simulink model "Basic_DMT"  (R2014b)
settings: Solver=FixedStepDiscrete  SolverMode=SingleTasking  StartTime=0.0  StopTime=25e-6-14e-9*24  RelTol=1e-3
PreLoadFcn:
  | userName = getenv('UserName');
  | 
  | if strcmp(userName,'Tim')
  | cd C:\Users\Tim\Documents\GitHub\MA_1\Basic_DMT
  | else
  | cd C:\Users\Tim-UML\Documents\GitHub\MA_1\Basic_DMT
  | end
InitFcn:
  | userName = getenv('UserName');
  | 
  | if strcmp(userName,'Tim')
  | cd C:\Users\Tim\Documents\GitHub\MA_1\Basic_DMT
  | else
  | cd C:\Users\Tim-UML\Documents\GitHub\MA_1\Basic_DMT
  | end
values from neighbouring files (symbols this model uses):
  a0 = 0.21194908595403703    (= 0.211949085954)    [initScript.m]
  a1 = 0.576101828091926    (= 0.576101828092)    [initScript.m]
  a2 = a0    (= 0.211949085954)    [initScript.m]
  beta = 1    [initScript.m]
  bitPerSymb = 4    [initScript.m]
  chanDownFact = Tchan/SystemPeriod    [initScript.m]
  fftLen = 16    [initScript.m]
  fftLenActive = fftLenDMT    (= 32)    [initScript.m]
  fftLenDMT = 2*fftLen    (= 32)    [initScript.m]
  GI_Active = GI_LenDMT    (= 0)    [initScript.m]
  GI_Len = 0    [initScript.m]
  GI_LenDMT = 0    [initScript.m]
  M = log2(fftLen)    [initScript.m]
  sysgenSystemPeriod = 4e-9    (= 4e-09)    [initScript.m]
  SystemPeriod = 4e-9    (= 4e-09)    [initScript.m]
  upsampleFactor = 1    [initScript.m]
  usedSubCar = 14    [initScript.m]
undefined symbols (not defined in the file or in its folder): bitCount, get, modu_mode, Tb, Ts
libraries: xbsIndex_r4 x822, commdigbbndam3 x59, simulink x42, dspsigops x7, commrandsrc2 x6, dspbuff3 x4, dspxfrm3 x3, dspswit3 x2, commseqgen2 x1, dsparch4 x1, commutil2 x1, dspsnks4 x1
(part 7 of 10)

== system Basic_DMT/IFFTaPIS/Guard_Interval/Set_GI_DMT ==
  note: 13
  note: max count == fftLen+GI_Len-1?
      | initial value== fftLen-1?
  In1 : Inport
  Complex to Real-Imag : ComplexToRealImag
  Constant : Constant
  Counter : dspswit3/Counter  Direction=Up  CountEvent=Free running  CounterSize=User defined  MaxCount=fftLenDMT+GI_LenDMT-1  InitialCount=32  Output=Count  HitValue=5  ResetInput=off  SamplesPerFrame=1  Ts=Tb*usedSubCar*bitPerSymb/fftLenDMT*beta  CntDtype=double  HitDtype=Logical
  Delay : Delay  DelayLength=53  InitialCondition=0
  Demux : Demux  Outputs=32
  Fcn : Fcn  Expr=u>fftLenDMT-1
  From Workspace : FromWorkspace  Commented=on  VariableName=sig_dmt_GI  SampleTime=1.12e-6  Interpolate=off  OutputAfterFinalValue=Setting to zero
  Mux : Mux  Inputs=40
  Scope : Scope  NumInputPorts=2
      settings: YMin=-5~-5  YMax=5~5  SaveName=ScopeData31
  Spectrum Analyzer1 : SpectrumAnalyzer  Commented=on
  Terminator : Terminator
  To Workspace : ToWorkspace  Commented=on  VariableName=sig_dmt_GI  SaveFormat=Structure  SampleTime=-1
  Unbuffer1 : Unbuffer  SampleBasedProcessing=Same as frame based
  Out1 : Outport
  pop : Outport  Port=2
  wires:
  In1/1 -> Demux/1
  Fcn/1 -> Scope/2
  Mux/1 -> To Workspace/1, Unbuffer1/1
  Complex to Real-Imag/1 -> Scope/1
  Complex to Real-Imag/2 -> Terminator/1
  Counter/1 -> Fcn/1
  Delay/1 -> Out1/1
  Demux/32 -> Mux/8, Mux/40
  Demux/31 -> Mux/7, Mux/39
  Demux/30 -> Mux/6, Mux/38
  Demux/29 -> Mux/5, Mux/37
  Demux/28 -> Mux/4, Mux/36
  Demux/27 -> Mux/3, Mux/35
  Demux/26 -> Mux/2, Mux/34
  Demux/25 -> Mux/1, Mux/33
  Demux/24 -> Mux/32
  Demux/23 -> Mux/31
  Demux/22 -> Mux/30
  Demux/21 -> Mux/29
  Demux/20 -> Mux/28
  Demux/19 -> Mux/27
  Demux/18 -> Mux/26
  Demux/17 -> Mux/25
  Demux/16 -> Mux/24
  Demux/15 -> Mux/23
  Demux/14 -> Mux/22
  Demux/13 -> Mux/21
  Demux/12 -> Mux/20
  Demux/11 -> Mux/19
  Demux/10 -> Mux/18
  Demux/9 -> Mux/17
  Demux/8 -> Mux/16
  Demux/7 -> Mux/15
  Demux/6 -> Mux/14
  Demux/5 -> Mux/13
  Demux/4 -> Mux/12
  Demux/3 -> Mux/11
  Demux/2 -> Mux/10
  Demux/1 -> Mux/9
  Unbuffer1/1 -> Delay/1, Complex to Real-Imag/1
  From Workspace/1 -> Spectrum Analyzer1/1
  Constant/1 -> pop/1

== system Basic_DMT/IFFTaPIS/Guard_Interval/Set_GI_OFDM ==
  note: 13
  note: max count == fftLen+GI_Len-1?
      | initial value== fftLen-1?
  note: 33
  In1 : Inport
  Complex to Real-Imag : ComplexToRealImag  Commented=on
  Complex to Real-Imag1 : ComplexToRealImag
  Complex to Real-Imag2 : ComplexToRealImag
  Counter : dspswit3/Counter  Commented=on  Direction=Up  CountEvent=Free running  CounterSize=User defined  MaxCount=19  InitialCount=16  Output=Count  HitValue=5  ResetInput=off  SamplesPerFrame=1  Ts=Tb*usedSubCar*bitPerSymb/fftLen*beta  CntDtype=double  HitDtype=Logical
  Data Store Memory : DataStoreMemory  DataStoreName=state  OutDataTypeStr=double
  Data Store Memory2 : DataStoreMemory  DataStoreName=loopCount  OutDataTypeStr=double
  Delay : Delay  Commented=on  DelayLength=33  InitialCondition=0
  Delay{1..17} (17 alike) : Delay  DelayLength=1  InitialCondition=0
  Delay18 : Delay  Commented=through  DelayLength=33  InitialCondition=0
  Delay19 : Delay  Commented=through  DelayLength=33  InitialCondition=0
  Demux1 : Demux  Commented=on  Outputs=16
  Fcn : Fcn  Commented=on  Expr=u>fftLen-1
  MATLAB Function : MATLAB Function  TreatAsAtomicUnit=on  SystemSampleTime=SystemPeriod*bitPerSymb*usedSubCar/fftLenActive
  Mux1 : Mux  Commented=on  Inputs=20
  Scope : Scope  Commented=on  NumInputPorts=2
      settings: YMin=-5~-5  YMax=5~5  SaveName=ScopeData31
  Scope1 : Scope  NumInputPorts=3
      settings: YMin=-5~-5~-5  YMax=5~5~5  SaveName=ScopeData69
  Terminator : Terminator  Commented=on
  Unbuffer1 : Unbuffer  Commented=on  SampleBasedProcessing=Same as frame based
  Unbuffer2 : Unbuffer  SampleBasedProcessing=Same as frame based
  Out1 : Outport
  pop : Outport  Port=2
  wires:
  Fcn/1 -> Scope/2
  Unbuffer1/1 -> Complex to Real-Imag/1, Delay/1
  Complex to Real-Imag/1 -> Scope/1
  Complex to Real-Imag/2 -> Terminator/1
  Counter/1 -> Fcn/1
  Demux1/8 -> Mux1/12
  Demux1/7 -> Mux1/11
  Demux1/6 -> Mux1/10
  Demux1/5 -> Mux1/9
  Demux1/4 -> Mux1/8
  Demux1/3 -> Mux1/7
  Demux1/2 -> Mux1/6
  Demux1/1 -> Mux1/5
  Mux1/1 -> Unbuffer1/1
  Demux1/9 -> Mux1/13
  Demux1/10 -> Mux1/14
  Demux1/11 -> Mux1/15
  Demux1/12 -> Mux1/16
  Demux1/13 -> Mux1/1, Mux1/17
  Demux1/14 -> Mux1/2, Mux1/18
  Demux1/15 -> Mux1/3, Mux1/19
  Demux1/16 -> Mux1/4, Mux1/20
  MATLAB Function/2(o1) -> Delay1/1
  MATLAB Function/3(o2) -> Delay2/1
  MATLAB Function/4(o3) -> Delay3/1
  MATLAB Function/5(o4) -> Delay4/1
  MATLAB Function/9(o8) -> Delay8/1
  MATLAB Function/8(o7) -> Delay7/1
  MATLAB Function/7(o6) -> Delay6/1
  MATLAB Function/6(o5) -> Delay5/1
  MATLAB Function/13(o12) -> Delay12/1
  MATLAB Function/12(o11) -> Delay11/1
  MATLAB Function/11(o10) -> Delay10/1
  MATLAB Function/10(o9) -> Delay9/1
  MATLAB Function/14(o13) -> Delay13/1
  MATLAB Function/15(o14) -> Delay14/1
  MATLAB Function/16(o15) -> Delay15/1
  MATLAB Function/17(o16) -> Delay16/1
  Delay16/1 -> MATLAB Function/17(i16)
  Delay15/1 -> MATLAB Function/16(i15)
  Delay14/1 -> MATLAB Function/15(i14)
  Delay13/1 -> MATLAB Function/14(i13)
  Delay12/1 -> MATLAB Function/13(i12)
  Delay11/1 -> MATLAB Function/12(i11)
  Delay10/1 -> MATLAB Function/11(i10)
  Delay9/1 -> MATLAB Function/10(i9)
  Delay8/1 -> MATLAB Function/9(i8)
  Delay7/1 -> MATLAB Function/8(i7)
  Delay6/1 -> MATLAB Function/7(i6)
  Delay5/1 -> MATLAB Function/6(i5)
  Delay4/1 -> MATLAB Function/5(i4)
  Delay3/1 -> MATLAB Function/4(i3)
  Delay2/1 -> MATLAB Function/3(i2)
  Delay1/1 -> MATLAB Function/2(i1)
  Unbuffer2/1 -> Delay17/1
  In1/1 -> Unbuffer2/1
  MATLAB Function/18(pop) -> Scope1/3, Delay19/1
  Complex to Real-Imag1/1 -> Scope1/2
  Complex to Real-Imag2/1 -> Scope1/1
  Delay17/1 -> Complex to Real-Imag2/1, MATLAB Function/1(inp)
  MATLAB Function/1(out) -> Delay18/1, Complex to Real-Imag1/1
  Delay18/1 -> Out1/1
  Delay19/1 -> pop/1

== system Basic_DMT/IFFTaPIS/upsample/upsample_No ==
  In1 : Inport
  Out1 : Outport
  wires:
  In1/1 -> Out1/1

== system Basic_DMT/IFFTaPIS/upsample/upsample_yes ==
  In1 : Inport
  Complex to Real-Imag : ComplexToRealImag
  Complex to Real-Imag1 : ComplexToRealImag
  Scope3 : Scope  NumInputPorts=4
      settings: YMin=-10~-8~-5~-5  YMax=8~8~5~5  SaveName=ScopeData38
  Unbuffer : Unbuffer  SampleBasedProcessing=Same as frame based
  Unbuffer1 : Unbuffer  SampleBasedProcessing=Same as frame based
  Upsample1 : dspsigops/Upsample  N=upsampleFactor  phase=0  InputProcessing=Columns as channels (frame based)  RateOptions=Enforce single-rate processing  ic=0  mode=Unused parameter value
  Out1 : Outport
  wires:
  In1/1 -> Unbuffer1/1, Upsample1/1
  Upsample1/1 -> Unbuffer/1, Out1/1
  Complex to Real-Imag/1 -> Scope3/1
  Complex to Real-Imag/2 -> Scope3/3
  Complex to Real-Imag1/1 -> Scope3/2
  Complex to Real-Imag1/2 -> Scope3/4
  Unbuffer/1 -> Complex to Real-Imag/1
  Unbuffer1/1 -> Complex to Real-Imag1/1

== system Basic_DMT/Modulation/Bit_Mapping_P1/16_QAM ==
  In1 : Inport
  Enable : EnablePort
  Rect_QAM_Mod : commdigbbndam3/Rectangular QAM Modulator Baseband  M=16  InType=Bit  Enc=Gray  Mapping=[0:15]  PowType=Min. distance between symbols  MinDist=2  AvgPow=1  PeakPow=1  Ph=0  outDtype=double  outWordLen=16  outUDDataType=sfix(16)  outFracLenMode=User-defined  outFracLen=13
  Out1 : Outport
  wires:
  Rect_QAM_Mod/1 -> Out1/1
  In1/1 -> Rect_QAM_Mod/1

== system Basic_DMT/Modulation/Bit_Mapping_P1/256_QAM ==
  In1 : Inport
  Enable : EnablePort
  Rect_QAM_Mod : commdigbbndam3/Rectangular QAM Modulator Baseband  M=16  InType=Bit  Enc=Gray  Mapping=[0:15]  PowType=Min. distance between symbols  MinDist=2  AvgPow=1  PeakPow=1  Ph=0  outDtype=double  outWordLen=16  outUDDataType=sfix(16)  outFracLenMode=User-defined  outFracLen=13
  Out1 : Outport
  wires:
  Rect_QAM_Mod/1 -> Out1/1
  In1/1 -> Rect_QAM_Mod/1

== system Basic_DMT/Modulation/Bit_Mapping_P10/16_QAM ==
  In1 : Inport
  Enable : EnablePort
  Rect_QAM_Mod : commdigbbndam3/Rectangular QAM Modulator Baseband  M=16  InType=Bit  Enc=Gray  Mapping=[0:15]  PowType=Min. distance between symbols  MinDist=2  AvgPow=1  PeakPow=1  Ph=0  outDtype=double  outWordLen=16  outUDDataType=sfix(16)  outFracLenMode=User-defined  outFracLen=13
  Out1 : Outport
  wires:
  Rect_QAM_Mod/1 -> Out1/1
  In1/1 -> Rect_QAM_Mod/1

== system Basic_DMT/Modulation/Bit_Mapping_P10/256_QAM ==
  In1 : Inport
  Enable : EnablePort
  Rect_QAM_Mod : commdigbbndam3/Rectangular QAM Modulator Baseband  M=16  InType=Bit  Enc=Gray  Mapping=[0:15]  PowType=Min. distance between symbols  MinDist=2  AvgPow=1  PeakPow=1  Ph=0  outDtype=double  outWordLen=16  outUDDataType=sfix(16)  outFracLenMode=User-defined  outFracLen=13
  Out1 : Outport
  wires:
  Rect_QAM_Mod/1 -> Out1/1
  In1/1 -> Rect_QAM_Mod/1

== system Basic_DMT/Modulation/Bit_Mapping_P11/16_QAM ==
  In1 : Inport
  Enable : EnablePort
  Rect_QAM_Mod : commdigbbndam3/Rectangular QAM Modulator Baseband  M=16  InType=Bit  Enc=Gray  Mapping=[0:15]  PowType=Min. distance between symbols  MinDist=2  AvgPow=1  PeakPow=1  Ph=0  outDtype=double  outWordLen=16  outUDDataType=sfix(16)  outFracLenMode=User-defined  outFracLen=13
  Out1 : Outport
  wires:
  Rect_QAM_Mod/1 -> Out1/1
  In1/1 -> Rect_QAM_Mod/1

== system Basic_DMT/Modulation/Bit_Mapping_P11/256_QAM ==
  In1 : Inport
  Enable : EnablePort
  Rect_QAM_Mod : commdigbbndam3/Rectangular QAM Modulator Baseband  M=16  InType=Bit  Enc=Gray  Mapping=[0:15]  PowType=Min. distance between symbols  MinDist=2  AvgPow=1  PeakPow=1  Ph=0  outDtype=double  outWordLen=16  outUDDataType=sfix(16)  outFracLenMode=User-defined  outFracLen=13
  Out1 : Outport
  wires:
  Rect_QAM_Mod/1 -> Out1/1
  In1/1 -> Rect_QAM_Mod/1

== system Basic_DMT/Modulation/Bit_Mapping_P12/16_QAM ==
  In1 : Inport
  Enable : EnablePort
  Rect_QAM_Mod : commdigbbndam3/Rectangular QAM Modulator Baseband  M=16  InType=Bit  Enc=Gray  Mapping=[0:15]  PowType=Min. distance between symbols  MinDist=2  AvgPow=1  PeakPow=1  Ph=0  outDtype=double  outWordLen=16  outUDDataType=sfix(16)  outFracLenMode=User-defined  outFracLen=13
  Out1 : Outport
  wires:
  Rect_QAM_Mod/1 -> Out1/1
  In1/1 -> Rect_QAM_Mod/1

== system Basic_DMT/Modulation/Bit_Mapping_P12/256_QAM ==
  In1 : Inport
  Enable : EnablePort
  Rect_QAM_Mod : commdigbbndam3/Rectangular QAM Modulator Baseband  M=16  InType=Bit  Enc=Gray  Mapping=[0:15]  PowType=Min. distance between symbols  MinDist=2  AvgPow=1  PeakPow=1  Ph=0  outDtype=double  outWordLen=16  outUDDataType=sfix(16)  outFracLenMode=User-defined  outFracLen=13
  Out1 : Outport
  wires:
  Rect_QAM_Mod/1 -> Out1/1
  In1/1 -> Rect_QAM_Mod/1

== system Basic_DMT/Modulation/Bit_Mapping_P13/16_QAM ==
  In1 : Inport
  Enable : EnablePort
  Rect_QAM_Mod : commdigbbndam3/Rectangular QAM Modulator Baseband  M=16  InType=Bit  Enc=Gray  Mapping=[0:15]  PowType=Min. distance between symbols  MinDist=2  AvgPow=1  PeakPow=1  Ph=0  outDtype=double  outWordLen=16  outUDDataType=sfix(16)  outFracLenMode=User-defined  outFracLen=13
  Out1 : Outport
  wires:
  Rect_QAM_Mod/1 -> Out1/1
  In1/1 -> Rect_QAM_Mod/1

== system Basic_DMT/Modulation/Bit_Mapping_P13/256_QAM ==
  In1 : Inport
  Enable : EnablePort
  Rect_QAM_Mod : commdigbbndam3/Rectangular QAM Modulator Baseband  M=16  InType=Bit  Enc=Gray  Mapping=[0:15]  PowType=Min. distance between symbols  MinDist=2  AvgPow=1  PeakPow=1  Ph=0  outDtype=double  outWordLen=16  outUDDataType=sfix(16)  outFracLenMode=User-defined  outFracLen=13
  Out1 : Outport
  wires:
  Rect_QAM_Mod/1 -> Out1/1
  In1/1 -> Rect_QAM_Mod/1

== system Basic_DMT/Modulation/Bit_Mapping_P14/16_QAM ==
  In1 : Inport
  Enable : EnablePort
  Rect_QAM_Mod : commdigbbndam3/Rectangular QAM Modulator Baseband  M=16  InType=Bit  Enc=Gray  Mapping=[0:15]  PowType=Min. distance between symbols  MinDist=2  AvgPow=1  PeakPow=1  Ph=0  outDtype=double  outWordLen=16  outUDDataType=sfix(16)  outFracLenMode=User-defined  outFracLen=13
  Out1 : Outport
  wires:
  Rect_QAM_Mod/1 -> Out1/1
  In1/1 -> Rect_QAM_Mod/1

== system Basic_DMT/Modulation/Bit_Mapping_P14/256_QAM ==
  In1 : Inport
  Enable : EnablePort
  Rect_QAM_Mod : commdigbbndam3/Rectangular QAM Modulator Baseband  M=16  InType=Bit  Enc=Gray  Mapping=[0:15]  PowType=Min. distance between symbols  MinDist=2  AvgPow=1  PeakPow=1  Ph=0  outDtype=double  outWordLen=16  outUDDataType=sfix(16)  outFracLenMode=User-defined  outFracLen=13
  Out1 : Outport
  wires:
  Rect_QAM_Mod/1 -> Out1/1
  In1/1 -> Rect_QAM_Mod/1

== system Basic_DMT/Modulation/Bit_Mapping_P2/16_QAM ==
  In1 : Inport
  Enable : EnablePort
  Rect_QAM_Mod : commdigbbndam3/Rectangular QAM Modulator Baseband  M=16  InType=Bit  Enc=Gray  Mapping=[0:15]  PowType=Min. distance between symbols  MinDist=2  AvgPow=1  PeakPow=1  Ph=0  outDtype=double  outWordLen=16  outUDDataType=sfix(16)  outFracLenMode=User-defined  outFracLen=13
  Out1 : Outport
  wires:
  Rect_QAM_Mod/1 -> Out1/1
  In1/1 -> Rect_QAM_Mod/1

== system Basic_DMT/Modulation/Bit_Mapping_P2/256_QAM ==
  In1 : Inport
  Enable : EnablePort
  Rect_QAM_Mod : commdigbbndam3/Rectangular QAM Modulator Baseband  M=16  InType=Bit  Enc=Gray  Mapping=[0:15]  PowType=Min. distance between symbols  MinDist=2  AvgPow=1  PeakPow=1  Ph=0  outDtype=double  outWordLen=16  outUDDataType=sfix(16)  outFracLenMode=User-defined  outFracLen=13
  Out1 : Outport
  wires:
  Rect_QAM_Mod/1 -> Out1/1
  In1/1 -> Rect_QAM_Mod/1

== system Basic_DMT/Modulation/Bit_Mapping_P3/16_QAM ==
  In1 : Inport
  Enable : EnablePort
  Rect_QAM_Mod : commdigbbndam3/Rectangular QAM Modulator Baseband  M=16  InType=Bit  Enc=Gray  Mapping=[0:15]  PowType=Min. distance between symbols  MinDist=2  AvgPow=1  PeakPow=1  Ph=0  outDtype=double  outWordLen=16  outUDDataType=sfix(16)  outFracLenMode=User-defined  outFracLen=13
  Out1 : Outport
  wires:
  Rect_QAM_Mod/1 -> Out1/1
  In1/1 -> Rect_QAM_Mod/1

== system Basic_DMT/Modulation/Bit_Mapping_P3/256_QAM ==
  In1 : Inport
  Enable : EnablePort
  Rect_QAM_Mod : commdigbbndam3/Rectangular QAM Modulator Baseband  M=16  InType=Bit  Enc=Gray  Mapping=[0:15]  PowType=Min. distance between symbols  MinDist=2  AvgPow=1  PeakPow=1  Ph=0  outDtype=double  outWordLen=16  outUDDataType=sfix(16)  outFracLenMode=User-defined  outFracLen=13
  Out1 : Outport
  wires:
  Rect_QAM_Mod/1 -> Out1/1
  In1/1 -> Rect_QAM_Mod/1

== system Basic_DMT/Modulation/Bit_Mapping_P4/16_QAM ==
  In1 : Inport
  Enable : EnablePort
  Rect_QAM_Mod : commdigbbndam3/Rectangular QAM Modulator Baseband  M=16  InType=Bit  Enc=Gray  Mapping=[0:15]  PowType=Min. distance between symbols  MinDist=2  AvgPow=1  PeakPow=1  Ph=0  outDtype=double  outWordLen=16  outUDDataType=sfix(16)  outFracLenMode=User-defined  outFracLen=13
  Out1 : Outport
  wires:
  Rect_QAM_Mod/1 -> Out1/1
  In1/1 -> Rect_QAM_Mod/1

== system Basic_DMT/Modulation/Bit_Mapping_P4/256_QAM ==
  In1 : Inport
  Enable : EnablePort
  Rect_QAM_Mod : commdigbbndam3/Rectangular QAM Modulator Baseband  M=16  InType=Bit  Enc=Gray  Mapping=[0:15]  PowType=Min. distance between symbols  MinDist=2  AvgPow=1  PeakPow=1  Ph=0  outDtype=double  outWordLen=16  outUDDataType=sfix(16)  outFracLenMode=User-defined  outFracLen=13
  Out1 : Outport
  wires:
  Rect_QAM_Mod/1 -> Out1/1
  In1/1 -> Rect_QAM_Mod/1

== system Basic_DMT/Modulation/Bit_Mapping_P5/16_QAM ==
  In1 : Inport
  Enable : EnablePort
  Rect_QAM_Mod : commdigbbndam3/Rectangular QAM Modulator Baseband  M=16  InType=Bit  Enc=Gray  Mapping=[0:15]  PowType=Min. distance between symbols  MinDist=2  AvgPow=1  PeakPow=1  Ph=0  outDtype=double  outWordLen=16  outUDDataType=sfix(16)  outFracLenMode=User-defined  outFracLen=13
  Out1 : Outport
  wires:
  Rect_QAM_Mod/1 -> Out1/1
  In1/1 -> Rect_QAM_Mod/1

== system Basic_DMT/Modulation/Bit_Mapping_P5/256_QAM ==
  In1 : Inport
  Enable : EnablePort
  Rect_QAM_Mod : commdigbbndam3/Rectangular QAM Modulator Baseband  M=16  InType=Bit  Enc=Gray  Mapping=[0:15]  PowType=Min. distance between symbols  MinDist=2  AvgPow=1  PeakPow=1  Ph=0  outDtype=double  outWordLen=16  outUDDataType=sfix(16)  outFracLenMode=User-defined  outFracLen=13
  Out1 : Outport
  wires:
  Rect_QAM_Mod/1 -> Out1/1
  In1/1 -> Rect_QAM_Mod/1

== system Basic_DMT/Modulation/Bit_Mapping_P6/16_QAM ==
  In1 : Inport
  Enable : EnablePort
  Rect_QAM_Mod : commdigbbndam3/Rectangular QAM Modulator Baseband  M=16  InType=Bit  Enc=Gray  Mapping=[0:15]  PowType=Min. distance between symbols  MinDist=2  AvgPow=1  PeakPow=1  Ph=0  outDtype=double  outWordLen=16  outUDDataType=sfix(16)  outFracLenMode=User-defined  outFracLen=13
  Out1 : Outport
  wires:
  Rect_QAM_Mod/1 -> Out1/1
  In1/1 -> Rect_QAM_Mod/1

== system Basic_DMT/Modulation/Bit_Mapping_P6/256_QAM ==
  In1 : Inport
  Enable : EnablePort
  Rect_QAM_Mod : commdigbbndam3/Rectangular QAM Modulator Baseband  M=16  InType=Bit  Enc=Gray  Mapping=[0:15]  PowType=Min. distance between symbols  MinDist=2  AvgPow=1  PeakPow=1  Ph=0  outDtype=double  outWordLen=16  outUDDataType=sfix(16)  outFracLenMode=User-defined  outFracLen=13
  Out1 : Outport
  wires:
  Rect_QAM_Mod/1 -> Out1/1
  In1/1 -> Rect_QAM_Mod/1

== system Basic_DMT/Modulation/Bit_Mapping_P7/16_QAM ==
  In1 : Inport
  Enable : EnablePort
  Rect_QAM_Mod : commdigbbndam3/Rectangular QAM Modulator Baseband  M=16  InType=Bit  Enc=Gray  Mapping=[0:15]  PowType=Min. distance between symbols  MinDist=2  AvgPow=1  PeakPow=1  Ph=0  outDtype=double  outWordLen=16  outUDDataType=sfix(16)  outFracLenMode=User-defined  outFracLen=13
  Out1 : Outport
  wires:
  Rect_QAM_Mod/1 -> Out1/1
  In1/1 -> Rect_QAM_Mod/1

== system Basic_DMT/Modulation/Bit_Mapping_P7/256_QAM ==
  In1 : Inport
  Enable : EnablePort
  Rect_QAM_Mod : commdigbbndam3/Rectangular QAM Modulator Baseband  M=16  InType=Bit  Enc=Gray  Mapping=[0:15]  PowType=Min. distance between symbols  MinDist=2  AvgPow=1  PeakPow=1  Ph=0  outDtype=double  outWordLen=16  outUDDataType=sfix(16)  outFracLenMode=User-defined  outFracLen=13
  Out1 : Outport
  wires:
  Rect_QAM_Mod/1 -> Out1/1
  In1/1 -> Rect_QAM_Mod/1

== system Basic_DMT/Modulation/Bit_Mapping_P8/16_QAM ==
  In1 : Inport
  Enable : EnablePort
  Rect_QAM_Mod : commdigbbndam3/Rectangular QAM Modulator Baseband  M=16  InType=Bit  Enc=Gray  Mapping=[0:15]  PowType=Min. distance between symbols  MinDist=2  AvgPow=1  PeakPow=1  Ph=0  outDtype=double  outWordLen=16  outUDDataType=sfix(16)  outFracLenMode=User-defined  outFracLen=13
  Out1 : Outport
  wires:
  Rect_QAM_Mod/1 -> Out1/1
  In1/1 -> Rect_QAM_Mod/1

== system Basic_DMT/Modulation/Bit_Mapping_P8/256_QAM ==
  In1 : Inport
  Enable : EnablePort
  Rect_QAM_Mod : commdigbbndam3/Rectangular QAM Modulator Baseband  M=16  InType=Bit  Enc=Gray  Mapping=[0:15]  PowType=Min. distance between symbols  MinDist=2  AvgPow=1  PeakPow=1  Ph=0  outDtype=double  outWordLen=16  outUDDataType=sfix(16)  outFracLenMode=User-defined  outFracLen=13
  Out1 : Outport
  wires:
  Rect_QAM_Mod/1 -> Out1/1
  In1/1 -> Rect_QAM_Mod/1

== system Basic_DMT/Modulation/Bit_Mapping_P9/16_QAM ==
  In1 : Inport
  Enable : EnablePort
  Rect_QAM_Mod : commdigbbndam3/Rectangular QAM Modulator Baseband  M=16  InType=Bit  Enc=Gray  Mapping=[0:15]  PowType=Min. distance between symbols  MinDist=2  AvgPow=1  PeakPow=1  Ph=0  outDtype=double  outWordLen=16  outUDDataType=sfix(16)  outFracLenMode=User-defined  outFracLen=13
  Out1 : Outport
  wires:
  Rect_QAM_Mod/1 -> Out1/1
  In1/1 -> Rect_QAM_Mod/1

== system Basic_DMT/Modulation/Bit_Mapping_P9/256_QAM ==
  In1 : Inport
  Enable : EnablePort
  Rect_QAM_Mod : commdigbbndam3/Rectangular QAM Modulator Baseband  M=16  InType=Bit  Enc=Gray  Mapping=[0:15]  PowType=Min. distance between symbols  MinDist=2  AvgPow=1  PeakPow=1  Ph=0  outDtype=double  outWordLen=16  outUDDataType=sfix(16)  outFracLenMode=User-defined  outFracLen=13
  Out1 : Outport
  wires:
  Rect_QAM_Mod/1 -> Out1/1
  In1/1 -> Rect_QAM_Mod/1

== system Basic_DMT/SIPaFFT/Delay_Guard_Interval1/None ==
  In1 : Inport
  Out1 : Outport
  wires:
  In1/1 -> Out1/1

== system Basic_DMT/SIPaFFT/Delay_Guard_Interval1/Rem_GI ==
  In1 : Inport
  Delay : Delay  DelayLength=1  InitialCondition=0
  Out1 : Outport
  wires:
  In1/1 -> Delay/1
  Delay/1 -> Out1/1

== system Basic_DMT/SIPaFFT/Delay_Guard_Interval2/No_equal ==
  In1 : Inport
  In2 : Inport  Port=2
  In3 : Inport  Port=3
  In4 : Inport  Port=4
  In5 : Inport  Port=5
  In6 : Inport  Port=6
  In7 : Inport  Port=7
  In8 : Inport  Port=8
  In9 : Inport  Port=9
  In10 : Inport  Port=10
  In11 : Inport  Port=11
  In12 : Inport  Port=12
  In13 : Inport  Port=13
  In14 : Inport  Port=14
  In15 : Inport  Port=15
  In16 : Inport  Port=16
  Out1 : Outport
  Out2 : Outport  Port=2
  Out3 : Outport  Port=3
  Out4 : Outport  Port=4
  Out5 : Outport  Port=5
  Out6 : Outport  Port=6
  Out7 : Outport  Port=7
  Out8 : Outport  Port=8
  Out9 : Outport  Port=9
  Out10 : Outport  Port=10
  Out11 : Outport  Port=11
  Out12 : Outport  Port=12
  Out13 : Outport  Port=13
  Out14 : Outport  Port=14
  Out15 : Outport  Port=15
  Out16 : Outport  Port=16
  wires:
  In1/1 -> Out1/1
  In2/1 -> Out2/1
  In3/1 -> Out3/1
  In4/1 -> Out4/1
  In5/1 -> Out5/1
  In6/1 -> Out6/1
  In7/1 -> Out7/1
  In8/1 -> Out8/1
  In9/1 -> Out9/1
  In10/1 -> Out10/1
  In11/1 -> Out11/1
  In12/1 -> Out12/1
  In13/1 -> Out13/1
  In14/1 -> Out14/1
  In15/1 -> Out15/1
  In16/1 -> Out16/1

== system Basic_DMT/SIPaFFT/Delay_Guard_Interval2/Yes_equal ==
  In1 : Inport
  In2 : Inport  Port=2
  In3 : Inport  Port=3
  In4 : Inport  Port=4
  In5 : Inport  Port=5
  In6 : Inport  Port=6
  In7 : Inport  Port=7
  In8 : Inport  Port=8
  In9 : Inport  Port=9
  In10 : Inport  Port=10
  In11 : Inport  Port=11
  In12 : Inport  Port=12
  In13 : Inport  Port=13
  In14 : Inport  Port=14
  In15 : Inport  Port=15
  In16 : Inport  Port=16
  Gain1 : Gain  Gain=1/e9  OutDataTypeStr=Inherit: Same as input
  Gain10 : Gain  Gain=1/e12  OutDataTypeStr=Inherit: Same as input
  Gain11 : Gain  Gain=1/e13  OutDataTypeStr=Inherit: Same as input
  Gain12 : Gain  Gain=1/e14  OutDataTypeStr=Inherit: Same as input
  Gain13 : Gain  Gain=1/e15  OutDataTypeStr=Inherit: Same as input
  Gain14 : Gain  Gain=1/e16  OutDataTypeStr=Inherit: Same as input
  Gain15 : Gain  Gain=1/e1  OutDataTypeStr=Inherit: Same as input
  Gain2 : Gain  Gain=1/e10  OutDataTypeStr=Inherit: Same as input
  Gain3 : Gain  Gain=1/e3  OutDataTypeStr=Inherit: Same as input
  Gain32 : Gain  Gain=1/e2  OutDataTypeStr=Inherit: Same as input
  Gain4 : Gain  Gain=1/e4  OutDataTypeStr=Inherit: Same as input
  Gain5 : Gain  Gain=1/e5  OutDataTypeStr=Inherit: Same as input
  Gain6 : Gain  Gain=1/e6  OutDataTypeStr=Inherit: Same as input
  Gain7 : Gain  Gain=1/e7  OutDataTypeStr=Inherit: Same as input
  Gain8 : Gain  Gain=1/e8  OutDataTypeStr=Inherit: Same as input
  Gain9 : Gain  Gain=1/e11  OutDataTypeStr=Inherit: Same as input
  Out1 : Outport
  Out2 : Outport  Port=2
  Out3 : Outport  Port=3
  Out4 : Outport  Port=4
  Out5 : Outport  Port=5
  Out6 : Outport  Port=6
  Out7 : Outport  Port=7
  Out8 : Outport  Port=8
  Out9 : Outport  Port=9
  Out10 : Outport  Port=10
  Out11 : Outport  Port=11
  Out12 : Outport  Port=12
  Out13 : Outport  Port=13
  Out14 : Outport  Port=14
  Out15 : Outport  Port=15
  Out16 : Outport  Port=16
  wires:
  In1/1 -> Gain1/1
  In2/1 -> Gain2/1
  In3/1 -> Gain9/1
  In4/1 -> Gain10/1
  In5/1 -> Gain11/1
  In6/1 -> Gain12/1
  In7/1 -> Gain13/1
  In8/1 -> Gain14/1
  In9/1 -> Gain15/1
  In10/1 -> Gain32/1
  In11/1 -> Gain3/1
  In12/1 -> Gain4/1
  In13/1 -> Gain5/1
  In14/1 -> Gain6/1
  In15/1 -> Gain7/1
  In16/1 -> Gain8/1
  Gain1/1 -> Out1/1
  Gain2/1 -> Out2/1
  Gain9/1 -> Out3/1
  Gain10/1 -> Out4/1
  Gain11/1 -> Out5/1
  Gain12/1 -> Out6/1
  Gain13/1 -> Out7/1
  Gain14/1 -> Out8/1
  Gain15/1 -> Out9/1
  Gain32/1 -> Out10/1
  Gain3/1 -> Out11/1
  Gain4/1 -> Out12/1
  Gain5/1 -> Out13/1
  Gain6/1 -> Out14/1
  Gain7/1 -> Out15/1
  Gain8/1 -> Out16/1

== system Basic_DMT/SIPaFFT/Delay_upsample/Del_ups ==
  In1 : Inport
  Out1 : Outport
  wires:
  In1/1 -> Out1/1

== system Basic_DMT/SIPaFFT/Delay_upsample/Del_ups_GI ==
  note: 26
  In1 : Inport
  Delay : Delay  DelayLength=28  InitialCondition=0  InputProcessing=Columns as channels (frame based)
  Out1 : Outport
  wires:
  In1/1 -> Delay/1
  Delay/1 -> Out1/1

== system Basic_DMT/SIPaFFT/Delay_upsample/Delay_None ==
  In1 : Inport
  up_downsample : Delay  InitialCondition=0  InputProcessing=Columns as channels (frame based)
  Out1 : Outport
  wires:
  In1/1 -> up_downsample/1
  up_downsample/1 -> Out1/1

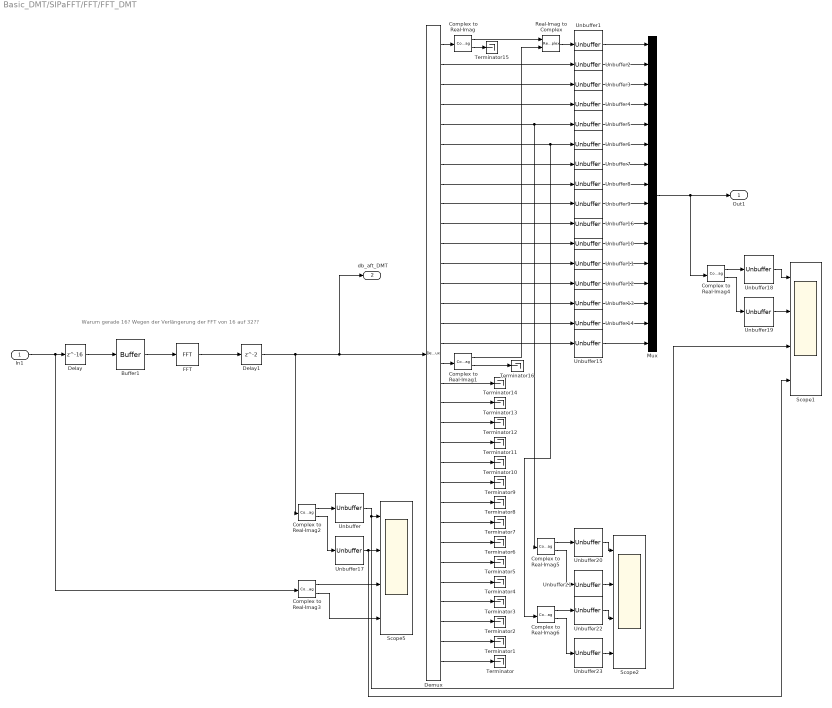
== system Basic_DMT/SIPaFFT/FFT/FFT_DMT ==
  note: Warum gerade 16? Wegen der Verlängerung der FFT von 16 auf 32??
  In1 : Inport
  Buffer1 : Buffer  N=32  TreatMby1Signals=One channel
  Complex to Real-Imag{,1..6} (7 alike) : ComplexToRealImag
  Delay : Delay  DelayLength=16  InitialCondition=0
  Delay1 : Delay  InitialCondition=0
  Demux : Demux  Outputs=32
  FFT : dspxfrm3/FFT  CompMethod=Table lookup  TableOpt=NEW  TableOptActive=Speed  BitRevOrder=off  InheritFFTLength=on  FFTLength=64  WrapInput=on  RowConvenienceOn=on  FFTImplementation=Auto  SkipNorm=on  firstCoeffDataTypeStr=Inherit: Same word length as input  firstCoeffLastDataTypeStr=Inherit: Same word length as input  outputMin=[]  outputMax=[]  roundingMode=Convergent  overflowMode=on
  Mux : Mux  Inputs=16
  Real-Imag to Complex : RealImagToComplex
  Scope1 : Scope  NumInputPorts=4
      settings: YMin=0~0~0~0  YMax=1~1~1~1  SaveName=ScopeData62
  Scope2 : Scope  NumInputPorts=4
      settings: YMin=-5~-5~-5~-5  YMax=5~5~5~5  SaveName=ScopeData64
  Scope5 : Scope  NumInputPorts=4
      settings: YMin=-5~-5~-5~-5  YMax=5~5~5~5  SaveName=ScopeData58
  Terminator{,1..16} (17 alike) : Terminator
  Unbuffer{,1..23} (24 alike) : Unbuffer  SampleBasedProcessing=Same as frame based
  Out1 : Outport
  db_aft_DMT : Outport  Port=2
  wires:
  In1/1 -> Delay/1, Complex to Real-Imag3/1
  Demux/8 -> Unbuffer8/1
  Demux/7 -> Unbuffer7/1
  Demux/6 -> Complex to Real-Imag6/1, Unbuffer6/1
  Demux/4 -> Unbuffer4/1
  Demux/3 -> Unbuffer3/1
  Demux/2 -> Unbuffer2/1
  Demux/1 -> Complex to Real-Imag/1
  Unbuffer1/1 -> Mux/1
  Unbuffer2/1 -> Mux/2
  Unbuffer3/1 -> Mux/3
  Unbuffer4/1 -> Mux/4
  Unbuffer5/1 -> Mux/5
  Unbuffer6/1 -> Mux/6
  Unbuffer7/1 -> Mux/7
  Unbuffer8/1 -> Mux/8
  Mux/1 -> Complex to Real-Imag4/1, Out1/1
  Demux/9 -> Unbuffer9/1
  Demux/10 -> Unbuffer16/1
  Demux/11 -> Unbuffer10/1
  Demux/12 -> Unbuffer11/1
  Demux/13 -> Unbuffer12/1
  Demux/14 -> Unbuffer13/1
  Demux/16 -> Unbuffer15/1
  Demux/15 -> Unbuffer14/1
  Unbuffer15/1 -> Mux/16
  Unbuffer14/1 -> Mux/15
  Unbuffer13/1 -> Mux/14
  Unbuffer12/1 -> Mux/13
  Unbuffer11/1 -> Mux/12
  Unbuffer10/1 -> Mux/11
  Unbuffer16/1 -> Mux/10
  Unbuffer9/1 -> Mux/9
  Demux/32 -> Terminator/1
  Demux/31 -> Terminator1/1
  Demux/30 -> Terminator2/1
  Demux/29 -> Terminator3/1
  Demux/25 -> Terminator7/1
  Demux/26 -> Terminator6/1
  Demux/27 -> Terminator5/1
  Demux/28 -> Terminator4/1
  Demux/21 -> Terminator11/1
  Demux/22 -> Terminator10/1
  Demux/23 -> Terminator9/1
  Demux/24 -> Terminator8/1
  Demux/18 -> Terminator14/1
  Demux/19 -> Terminator13/1
  Demux/20 -> Terminator12/1
  Buffer1/1 -> FFT/1
  Real-Imag to Complex/1 -> Unbuffer1/1
  Complex to Real-Imag/2 -> Terminator15/1
  Complex to Real-Imag/1 -> Real-Imag to Complex/1
  Demux/17 -> Complex to Real-Imag1/1
  Complex to Real-Imag1/1 -> Real-Imag to Complex/2
  Complex to Real-Imag1/2 -> Terminator16/1
  Unbuffer/1 -> Scope1/3, Scope5/1
  Complex to Real-Imag2/1 -> Unbuffer/1
  Complex to Real-Imag2/2 -> Unbuffer17/1
  Unbuffer17/1 -> Scope1/4, Scope5/2
  Complex to Real-Imag3/2 -> Scope5/4
  Complex to Real-Imag3/1 -> Scope5/3
  Unbuffer18/1 -> Scope1/1
  Complex to Real-Imag4/1 -> Unbuffer18/1
  Complex to Real-Imag4/2 -> Unbuffer19/1
  Unbuffer19/1 -> Scope1/2
  Complex to Real-Imag5/1 -> Unbuffer20/1
  Complex to Real-Imag5/2 -> Unbuffer21/1
  Unbuffer21/1 -> Scope2/2
  Unbuffer20/1 -> Scope2/1
  Complex to Real-Imag6/1 -> Unbuffer22/1
  Complex to Real-Imag6/2 -> Unbuffer23/1
  Unbuffer23/1 -> Scope2/4
  Unbuffer22/1 -> Scope2/3
  Demux/5 -> Complex to Real-Imag5/1, Unbuffer5/1
  FFT/1 -> Delay1/1
  Delay/1 -> Buffer1/1
  Delay1/1 -> db_aft_DMT/1, Demux/1, Complex to Real-Imag2/1

== system Basic_DMT/SIPaFFT/FFT/FFT_OFDM ==
  In1 : Inport
  Buffer : Buffer  N=16*upsampleFactor  TreatMby1Signals=One channel
  Constant : Constant
  FFT : dspxfrm3/FFT  CompMethod=Table lookup  TableOpt=NEW  TableOptActive=Speed  BitRevOrder=off  InheritFFTLength=on  FFTLength=64  WrapInput=on  RowConvenienceOn=on  FFTImplementation=Auto  SkipNorm=on  firstCoeffDataTypeStr=Inherit: Same word length as input  firstCoeffLastDataTypeStr=Inherit: Same word length as input  outputMin=[]  outputMax=[]  roundingMode=Convergent  overflowMode=on
  Real-Imag to Complex : RealImagToComplex
  Out1 : Outport
  db_aft_DMT : Outport  Port=2
  wires:
  In1/1 -> Buffer/1
  FFT/1 -> Out1/1
  Buffer/1 -> FFT/1
  Constant/1 -> Real-Imag to Complex/2, Real-Imag to Complex/1
  Real-Imag to Complex/1 -> db_aft_DMT/1

== system Basic_DMT/SIPaFFT/Remove_Guard_Interval/No_GI ==
  In1 : Inport
  Out1 : Outport
  wires:
  In1/1 -> Out1/1

== system Basic_DMT/SIPaFFT/Remove_Guard_Interval/Rem_GI_DMT ==
  note: 16
  note: 7
  In1 : Inport
  Buffer : Buffer  N=40  TreatMby1Signals=One channel
  Delay : Delay  DelayLength=7  InitialCondition=0
  Delay1 : Delay  DelayLength=16  InitialCondition=0
  Demux : Demux  Outputs=40
  Mux : Mux  Inputs=32
  Terminator{,1..7} (8 alike) : Terminator
  Unbuffer{,1..32} (33 alike) : Unbuffer  SampleBasedProcessing=Same as frame based
  Out1 : Outport
  wires:
  In1/1 -> Delay/1
  Buffer/1 -> Demux/1
  Mux/1 -> Unbuffer32/1
  Delay/1 -> Buffer/1
  Demux/40 -> Unbuffer31/1
  Demux/39 -> Unbuffer30/1
  Demux/38 -> Unbuffer29/1
  Demux/37 -> Unbuffer28/1
  Demux/36 -> Unbuffer27/1
  Demux/35 -> Unbuffer26/1
  Demux/34 -> Unbuffer25/1
  Demux/33 -> Unbuffer24/1
  Demux/32 -> Unbuffer23/1
  Demux/31 -> Unbuffer22/1
  Demux/30 -> Unbuffer21/1
  Demux/29 -> Unbuffer20/1
  Demux/28 -> Unbuffer19/1
  Demux/27 -> Unbuffer18/1
  Demux/26 -> Unbuffer17/1
  Demux/25 -> Unbuffer16/1
  Demux/24 -> Unbuffer15/1
  Demux/23 -> Unbuffer14/1
  Demux/22 -> Unbuffer13/1
  Demux/21 -> Unbuffer12/1
  Demux/20 -> Unbuffer11/1
  Demux/19 -> Unbuffer10/1
  Demux/18 -> Unbuffer9/1
  Demux/17 -> Unbuffer8/1
  Demux/16 -> Unbuffer7/1
  Demux/15 -> Unbuffer6/1
  Demux/14 -> Unbuffer5/1
  Demux/13 -> Unbuffer4/1
  Demux/12 -> Unbuffer3/1
  Demux/11 -> Unbuffer2/1
  Demux/10 -> Unbuffer1/1
  Demux/9 -> Unbuffer/1
  Unbuffer/1 -> Mux/1
  Unbuffer1/1 -> Mux/2
  Unbuffer2/1 -> Mux/3
  Unbuffer3/1 -> Mux/4
  Unbuffer4/1 -> Mux/5
  Unbuffer5/1 -> Mux/6
  Unbuffer6/1 -> Mux/7
  Unbuffer7/1 -> Mux/8
  Unbuffer8/1 -> Mux/9
  Unbuffer9/1 -> Mux/10
  Unbuffer10/1 -> Mux/11
  Unbuffer11/1 -> Mux/12
  Unbuffer12/1 -> Mux/13
  Unbuffer13/1 -> Mux/14
  Unbuffer14/1 -> Mux/15
  Unbuffer15/1 -> Mux/16
  Unbuffer16/1 -> Mux/17
  Unbuffer17/1 -> Mux/18
  Unbuffer18/1 -> Mux/19
  Unbuffer19/1 -> Mux/20
  Unbuffer20/1 -> Mux/21
  Unbuffer21/1 -> Mux/22
  Unbuffer22/1 -> Mux/23
  Unbuffer23/1 -> Mux/24
  Unbuffer24/1 -> Mux/25
  Unbuffer25/1 -> Mux/26
  Unbuffer26/1 -> Mux/27
  Unbuffer27/1 -> Mux/28
  Unbuffer28/1 -> Mux/29
  Unbuffer29/1 -> Mux/30
  Unbuffer30/1 -> Mux/31
  Unbuffer31/1 -> Mux/32
  Demux/8 -> Terminator/1
  Demux/7 -> Terminator1/1
  Demux/6 -> Terminator2/1
  Demux/5 -> Terminator3/1
  Demux/4 -> Terminator4/1
  Demux/3 -> Terminator5/1
  Demux/2 -> Terminator6/1
  Demux/1 -> Terminator7/1
  Unbuffer32/1 -> Delay1/1
  Delay1/1 -> Out1/1

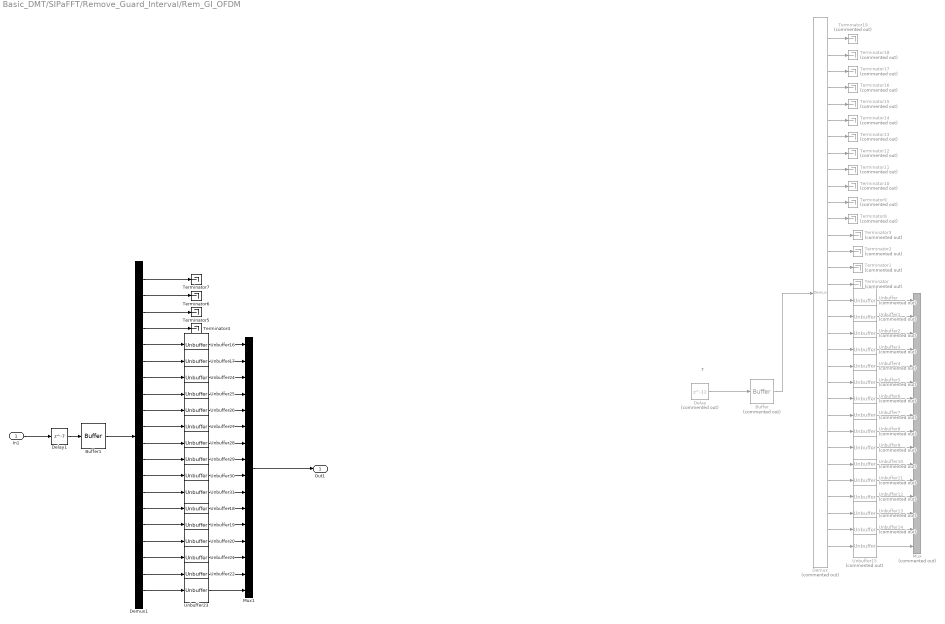
== system Basic_DMT/SIPaFFT/Remove_Guard_Interval/Rem_GI_OFDM ==
  note: 7
  In1 : Inport
  Buffer : Buffer  Commented=on  N=32  TreatMby1Signals=One channel
  Buffer1 : Buffer  N=fftLen+GI_Len  TreatMby1Signals=One channel
  Delay : Delay  Commented=on  DelayLength=11  InitialCondition=0
  Delay1 : Delay  DelayLength=7  InitialCondition=0
  Demux : Demux  Commented=on  Outputs=32
  Demux1 : Demux  Outputs=fftLen+GI_Len
  Mux : Mux  Commented=on  Inputs=16
  Mux1 : Mux  Inputs=16
  Terminator{,1..3,8..19} (16 alike) : Terminator  Commented=on
  Terminator{4..7} (4 alike) : Terminator
  Unbuffer{,1..15} (16 alike) : Unbuffer  Commented=on  SampleBasedProcessing=Same as frame based
  Unbuffer{16..31} (16 alike) : Unbuffer  SampleBasedProcessing=Same as frame based
  Out1 : Outport
  wires:
  In1/1 -> Delay1/1
  Demux1/12 -> Unbuffer29/1
  Demux1/11 -> Unbuffer28/1
  Demux1/10 -> Unbuffer27/1
  Demux1/9 -> Unbuffer26/1
  Demux1/8 -> Unbuffer25/1
  Demux1/7 -> Unbuffer24/1
  Demux1/6 -> Unbuffer17/1
  Demux1/5 -> Unbuffer16/1
  Demux1/4 -> Terminator4/1
  Demux1/3 -> Terminator5/1
  Demux1/2 -> Terminator6/1
  Demux1/1 -> Terminator7/1
  Unbuffer16/1 -> Mux1/1
  Unbuffer17/1 -> Mux1/2
  Unbuffer24/1 -> Mux1/3
  Unbuffer25/1 -> Mux1/4
  Unbuffer26/1 -> Mux1/5
  Unbuffer27/1 -> Mux1/6
  Unbuffer28/1 -> Mux1/7
  Unbuffer29/1 -> Mux1/8
  Buffer1/1 -> Demux1/1
  Mux1/1 -> Out1/1
  Delay1/1 -> Buffer1/1
  Demux1/13 -> Unbuffer30/1
  Demux1/14 -> Unbuffer31/1
  Demux1/15 -> Unbuffer18/1
  Demux1/16 -> Unbuffer19/1
  Demux1/17 -> Unbuffer20/1
  Demux1/18 -> Unbuffer21/1
  Demux1/20 -> Unbuffer23/1
  Demux1/19 -> Unbuffer22/1
  Unbuffer23/1 -> Mux1/16
  Unbuffer22/1 -> Mux1/15
  Unbuffer21/1 -> Mux1/14
  Unbuffer20/1 -> Mux1/13
  Unbuffer19/1 -> Mux1/12
  Unbuffer18/1 -> Mux1/11
  Unbuffer31/1 -> Mux1/10
  Unbuffer30/1 -> Mux1/9
  Unbuffer/1 -> Mux/1
  Unbuffer1/1 -> Mux/2
  Unbuffer2/1 -> Mux/3
  Unbuffer3/1 -> Mux/4
  Unbuffer4/1 -> Mux/5
  Unbuffer5/1 -> Mux/6
  Unbuffer6/1 -> Mux/7
  Unbuffer7/1 -> Mux/8
  Buffer/1 -> Demux/1
  Delay/1 -> Buffer/1
  Unbuffer15/1 -> Mux/16
  Unbuffer14/1 -> Mux/15
  Unbuffer13/1 -> Mux/14
  Unbuffer12/1 -> Mux/13
  Unbuffer11/1 -> Mux/12
  Unbuffer10/1 -> Mux/11
  Unbuffer9/1 -> Mux/10
  Unbuffer8/1 -> Mux/9
  Demux/32 -> Unbuffer15/1
  Demux/31 -> Unbuffer14/1
  Demux/30 -> Unbuffer13/1
  Demux/29 -> Unbuffer12/1
  Demux/28 -> Unbuffer11/1
  Demux/27 -> Unbuffer10/1
  Demux/26 -> Unbuffer9/1
  Demux/25 -> Unbuffer8/1
  Demux/24 -> Unbuffer7/1
  Demux/23 -> Unbuffer6/1
  Demux/22 -> Unbuffer5/1
  Demux/21 -> Unbuffer4/1
  Demux/20 -> Unbuffer3/1
  Demux/19 -> Unbuffer2/1
  Demux/18 -> Unbuffer1/1
  Demux/17 -> Unbuffer/1
  Demux/16 -> Terminator/1
  Demux/15 -> Terminator1/1
  Demux/14 -> Terminator2/1
  Demux/13 -> Terminator3/1
  Demux/12 -> Terminator8/1
  Demux/11 -> Terminator9/1
  Demux/10 -> Terminator10/1
  Demux/9 -> Terminator11/1
  Demux/8 -> Terminator12/1
  Demux/7 -> Terminator13/1
  Demux/6 -> Terminator14/1
  Demux/5 -> Terminator15/1
  Demux/4 -> Terminator16/1
  Demux/3 -> Terminator17/1
  Demux/2 -> Terminator18/1
  Demux/1 -> Terminator19/1

== system Basic_DMT/SIPaFFT/downsample/No_downsample ==
  In1 : Inport
  Out1 : Outport
  wires:
  In1/1 -> Out1/1

== system Basic_DMT/SIPaFFT/downsample/Yes_downsample ==
  In1 : Inport
  Complex to Real-Imag : ComplexToRealImag
  Complex to Real-Imag1 : ComplexToRealImag
  Delay19 : Delay  DelayLength=32+96  InitialCondition=0  InputProcessing=Columns as channels (frame based)
  Downsample : dspsigops/Downsample  N=upsampleFactor  phase=0  InputProcessing=Columns as channels (frame based)  RateOptions=Allow multirate processing  smode=Allow multirate  fmode=Maintain input frame size  ic=0
  Scope3 : Scope  NumInputPorts=4
      settings: YMin=-10~-8~-5~-5  YMax=8~8~5~5  SaveName=ScopeData47
  Unbuffer : Unbuffer  SampleBasedProcessing=Same as frame based
  Unbuffer1 : Unbuffer  SampleBasedProcessing=Same as frame based
  Out1 : Outport
  wires:
  In1/1 -> Delay19/1, Downsample/1
  Complex to Real-Imag/1 -> Scope3/1
  Complex to Real-Imag/2 -> Scope3/3
  Complex to Real-Imag1/1 -> Scope3/2
  Complex to Real-Imag1/2 -> Scope3/4
  Unbuffer1/1 -> Complex to Real-Imag1/1
  Unbuffer/1 -> Complex to Real-Imag/1
  Delay19/1 -> Unbuffer1/1
  Downsample/1 -> Out1/1, Unbuffer/1

== system Basic_DMT/Sysgen_Channel/Yes_Channel/TP_2nd_ord ==
  Re1 : Inport
  Im1 : Inport  Port=2
  AddSub{4..7} (4 alike) : xbsIndex_r4/AddSub  mode=Addition  use_carryin=off  use_carryout=off  en=off  latency=0  precision=User Defined  arith_type="Signed  (2's comp)"  n_bits=bitCount+(log2(fftLen)+1)  bin_pt=fracLen  quantization="Round  (unbiased: +/- Inf)"  overflow=Saturate  use_behavioral_HDL=off  hw_selection=Fabric  pipelined=off  dbl_ovrd=off  block_type=addsub
  CMult{8..15} (8 alike) : xbsIndex_r4/CMult  const=.5  gui_display_data_type=Fixed-point  const_n_bits=bitCount+(log2(fftLen)+1)  const_bin_pt=fracLen  float_type=Single  exp_bits=8  fraction_bits=24  en=off  latency=0  precision=User Defined  arith_type="Signed  (2's comp)"  n_bits=bitCount+(log2(fftLen)+1)  bin_pt=fracLen  quantization="Round  (unbiased: +/- Inf)"  overflow=Saturate  use_behavioral_HDL=off  mem_type=Distributed RAM  pipeline=off  dbl_ovrd=off  block_type=cmult
  Delay10 : xbsIndex_r4/Delay  rst=off  infoeditControl=Selection of Reset will increase slice count due to use of real FFs and instead of SRLs  en=off  latency=fftLen-1+GI_Len  reg_retiming=off  dbl_ovrd=off  block_type=delay
  Delay11 : xbsIndex_r4/Delay  rst=off  infoeditControl=Selection of Reset will increase slice count due to use of real FFs and instead of SRLs  en=off  latency=fftLen-1+GI_Len  reg_retiming=off  dbl_ovrd=off  block_type=delay
  Delay{6..9} (4 alike) : xbsIndex_r4/Delay  rst=off  infoeditControl=Selection of Reset will increase slice count due to use of real FFs and instead of SRLs  en=off  latency=1  reg_retiming=off  dbl_ovrd=off  block_type=delay
  Re_out1 : Outport
  Im_out1 : Outport  Port=2
  wires:
  AddSub6/1 -> CMult14/1, Delay9/1
  CMult14/1 -> AddSub7/2
  CMult12/1 -> AddSub5/2
  Delay10/1 -> Re_out1/1
  Delay8/1 -> CMult13/1
  AddSub7/1 -> Delay11/1
  Im1/1 -> CMult10/1, Delay7/1
  Delay7/1 -> CMult11/1
  AddSub5/1 -> Delay10/1
  CMult8/1 -> AddSub4/2
  CMult11/1 -> AddSub6/1
  AddSub4/1 -> CMult12/1, Delay8/1
  CMult10/1 -> AddSub6/2
  Delay9/1 -> CMult15/1
  Re1/1 -> CMult8/1, Delay6/1
  CMult15/1 -> AddSub7/1
  CMult13/1 -> AddSub5/1
  Delay11/1 -> Im_out1/1
  Delay6/1 -> CMult9/1
  CMult9/1 -> AddSub4/1

== system Basic_DMT/Sysgen_IFFTaPIS/Guard_Interval/No_GI ==
  Re_In : Inport
  Im_In : Inport  Port=2
  Re : Outport
  Im : Outport  Port=2
  wires:
  Im_In/1 -> Im/1
  Re_In/1 -> Re/1

== system Basic_DMT/Sysgen_IFFTaPIS/Guard_Interval/Set_GI_DMT ==
  note: 12
  Re_In : Inport
  Im_In : Inport  Port=2
  Concat : xbsIndex_r4/Concat  num_inputs=2  dbl_ovrd=off  block_type=concat
  Concat1 : xbsIndex_r4/Concat  num_inputs=2  dbl_ovrd=off  block_type=concat
  Delay : xbsIndex_r4/Delay  rst=off  infoeditControl=Selection of Reset will increase slice count due to use of real FFs and instead of SRLs  en=off  latency=12  reg_retiming=off  dbl_ovrd=off  block_type=delay
  Delay1 : xbsIndex_r4/Delay  rst=off  infoeditControl=Selection of Reset will increase slice count due to use of real FFs and instead of SRLs  en=off  latency=12  reg_retiming=off  dbl_ovrd=off  block_type=delay
  Parallel to Serial : xbsIndex_r4/Parallel to Serial  output_order=Most Significant Word First  arith_type="Signed  (2's comp)"  output_bits=(bitCount+(log2(fftLen)+1))  bin_pt=fracLen  rst=off  en=off  latency=1  dbl_ovrd=off  block_type=p2s
      settings: infoedit=Each sample presented at the input becomes several samples presented serially at the output.
  Parallel to Serial1 : xbsIndex_r4/Parallel to Serial  output_order=Most Significant Word First  arith_type="Signed  (2's comp)"  output_bits=(bitCount+(log2(fftLen)+1))  bin_pt=fracLen  rst=off  en=off  latency=1  dbl_ovrd=off  block_type=p2s
      settings: infoedit=Each sample presented at the input becomes several samples presented serially at the output.
  Serial to Parallel : xbsIndex_r4/Serial to Parallel  input_order=Most Significant Word First  arith_type=Unsigned  output_bits=(bitCount+(log2(fftLen)+1))*fftLenDMT  bin_pt=0  rst=off  en=off  latency=1  dbl_ovrd=off  block_type=s2p
      settings: infoedit=Groups of samples presented serially at the input become single samples presented at the output.
  Serial to Parallel1 : xbsIndex_r4/Serial to Parallel  input_order=Most Significant Word First  arith_type=Unsigned  output_bits=(bitCount+(log2(fftLen)+1))*fftLenDMT  bin_pt=0  rst=off  en=off  latency=1  dbl_ovrd=off  block_type=s2p
      settings: infoedit=Groups of samples presented serially at the input become single samples presented at the output.
  Slice : xbsIndex_r4/Slice  nbits=(bitCount+(log2(fftLen)+1))*GI_LenDMT  boolean_output=off  mode=Lower Bit Location + Width  bit1=0  base1=LSB of Input  bit0=0  base0=LSB of Input  dbl_ovrd=off  block_type=slice
  Slice1 : xbsIndex_r4/Slice  nbits=(bitCount+(log2(fftLen)+1))*fftLenDMT  boolean_output=off  mode=Lower Bit Location + Width  bit1=0  base1=LSB of Input  bit0=0  base0=LSB of Input  dbl_ovrd=off  block_type=slice
  Slice2 : xbsIndex_r4/Slice  nbits=(bitCount+(log2(fftLen)+1))*GI_LenDMT  boolean_output=off  mode=Lower Bit Location + Width  bit1=0  base1=LSB of Input  bit0=0  base0=LSB of Input  dbl_ovrd=off  block_type=slice
  Slice3 : xbsIndex_r4/Slice  nbits=(bitCount+(log2(fftLen)+1))*fftLenDMT  boolean_output=off  mode=Lower Bit Location + Width  bit1=0  base1=LSB of Input  bit0=0  base0=LSB of Input  dbl_ovrd=off  block_type=slice
  Re : Outport
  Im : Outport  Port=2
  wires:
  Re_In/1 -> Serial to Parallel/1
  Concat/1 -> Parallel to Serial/1
  Im_In/1 -> Serial to Parallel1/1
  Parallel to Serial/1 -> Delay/1
  Delay/1 -> Re/1
  Serial to Parallel/1 -> Slice/1, Slice1/1
  Concat1/1 -> Parallel to Serial1/1
  Parallel to Serial1/1 -> Delay1/1
  Serial to Parallel1/1 -> Slice2/1, Slice3/1
  Delay1/1 -> Im/1
  Slice/1 -> Concat/1
  Slice1/1 -> Concat/2
  Slice3/1 -> Concat1/2
  Slice2/1 -> Concat1/1

== system Basic_DMT/Sysgen_IFFTaPIS/Guard_Interval/Set_GI_OFDM ==
  note: Zusammenfügen mit DEMUX anstelle von P/S um die Rate zu erhalten?
      | Im MCODE block
  Re_In : Inport
  Im_In : Inport  Port=2
  Concat2 : xbsIndex_r4/Concat  num_inputs=2  dbl_ovrd=off  block_type=concat
  Concat3 : xbsIndex_r4/Concat  num_inputs=2  dbl_ovrd=off  block_type=concat
  Delay : xbsIndex_r4/Delay  rst=off  infoeditControl=Selection of Reset will increase slice count due to use of real FFs and instead of SRLs  en=off  latency=12  reg_retiming=off  dbl_ovrd=off  block_type=delay
  Delay1 : xbsIndex_r4/Delay  rst=off  infoeditControl=Selection of Reset will increase slice count due to use of real FFs and instead of SRLs  en=off  latency=12  reg_retiming=off  dbl_ovrd=off  block_type=delay
  Parallel to Serial : xbsIndex_r4/Parallel to Serial  output_order=Most Significant Word First  arith_type="Signed  (2's comp)"  output_bits=(bitCount+(log2(fftLen)+1))  bin_pt=fracLen  rst=off  en=off  latency=1  dbl_ovrd=off  block_type=p2s
      settings: infoedit=Each sample presented at the input becomes several samples presented serially at the output.
  Parallel to Serial1 : xbsIndex_r4/Parallel to Serial  output_order=Most Significant Word First  arith_type="Signed  (2's comp)"  output_bits=(bitCount+(log2(fftLen)+1))  bin_pt=fracLen  rst=off  en=off  latency=1  dbl_ovrd=off  block_type=p2s
      settings: infoedit=Each sample presented at the input becomes several samples presented serially at the output.
  Serial to Parallel : xbsIndex_r4/Serial to Parallel  input_order=Most Significant Word First  arith_type=Unsigned  output_bits=(bitCount+(log2(fftLen)+1))*fftLen  bin_pt=0  rst=off  en=off  latency=1  dbl_ovrd=off  block_type=s2p
      settings: infoedit=Groups of samples presented serially at the input become single samples presented at the output.
  Serial to Parallel1 : xbsIndex_r4/Serial to Parallel  input_order=Most Significant Word First  arith_type=Unsigned  output_bits=(bitCount+(log2(fftLen)+1))*fftLen  bin_pt=0  rst=off  en=off  latency=1  dbl_ovrd=off  block_type=s2p
      settings: infoedit=Groups of samples presented serially at the input become single samples presented at the output.
  Slice32 : xbsIndex_r4/Slice  nbits=(bitCount+(log2(fftLen)+1))*GI_Len  boolean_output=off  mode=Lower Bit Location + Width  bit1=0  base1=LSB of Input  bit0=0  base0=LSB of Input  dbl_ovrd=off  block_type=slice
  Slice33 : xbsIndex_r4/Slice  nbits=(bitCount+(log2(fftLen)+1))*fftLen  boolean_output=off  mode=Lower Bit Location + Width  bit1=0  base1=LSB of Input  bit0=0  base0=LSB of Input  dbl_ovrd=off  block_type=slice
  Slice34 : xbsIndex_r4/Slice  nbits=(bitCount+(log2(fftLen)+1))*GI_Len  boolean_output=off  mode=Lower Bit Location + Width  bit1=0  base1=LSB of Input  bit0=0  base0=LSB of Input  dbl_ovrd=off  block_type=slice
  Slice35 : xbsIndex_r4/Slice  nbits=(bitCount+(log2(fftLen)+1))*fftLen  boolean_output=off  mode=Lower Bit Location + Width  bit1=0  base1=LSB of Input  bit0=0  base0=LSB of Input  dbl_ovrd=off  block_type=slice
  Re : Outport
  Im : Outport  Port=2
  wires:
  Re_In/1 -> Serial to Parallel/1
  Im_In/1 -> Serial to Parallel1/1
  Parallel to Serial/1 -> Delay/1
  Concat2/1 -> Parallel to Serial1/1
  Parallel to Serial1/1 -> Delay1/1
  Delay/1 -> Re/1
  Delay1/1 -> Im/1
  Serial to Parallel1/1 -> Slice33/1, Slice32/1
  Serial to Parallel/1 -> Slice35/1, Slice34/1
  Slice32/1 -> Concat2/1
  Slice33/1 -> Concat2/2
  Slice35/1 -> Concat3/2
  Slice34/1 -> Concat3/1
  Concat3/1 -> Parallel to Serial/1
